simulink model "problem4"  (R2020a)
settings: Solver=ode15s  StartTime=0.0  StopTime=10.0  RelTol=1e-3
settings Model: Creator=HP  LastModifiedBy=HP

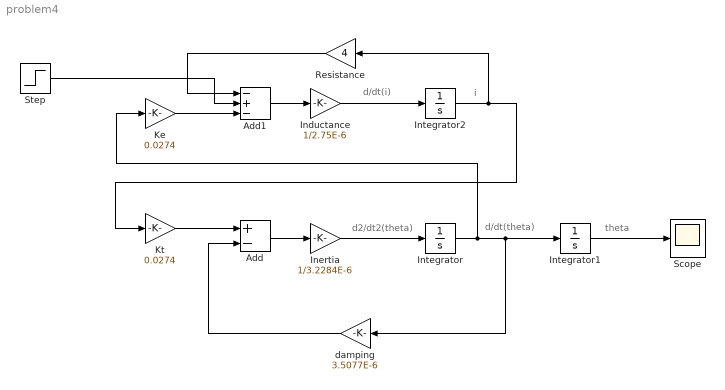
== system problem4 ==
  note: d/dt(theta)
  note: i
  note: d2/dt2(theta)
  note: d/dt(i)
  note: theta
  Add : Sum  Inputs=+-
  Add1 : Sum  Inputs=-+-
  Inductance : Gain  Gain=1/2.75E-6
  Inertia : Gain  Gain=1/3.2284E-6
  Integrator : Integrator
  Integrator1 : Integrator
  Integrator2 : Integrator
  Ke : Gain  Gain=0.0274
  Kt : Gain  Gain=0.0274
  Resistance : Gain  Gain=4
  Scope : Scope
  Step : Step  SampleTime=0
  damping : Gain  Gain=3.5077E-6
  wires:
  Inertia/1 -> Integrator/1
  Kt/1 -> Add/1
  Add1/1 -> Inductance/1
  Inductance/1 -> Integrator2/1
  Ke/1 -> Add1/3
  damping/1 -> Add/2
  Integrator1/1 -> Scope/1
  Step/1 -> Add1/2
  Integrator2/1 -> Resistance/1, Kt/1
  Integrator/1 -> Ke/1, damping/1, Integrator1/1
  Add/1 -> Inertia/1
  Resistance/1 -> Add1/1
